simulink model "Modelo_NL_PID_Y_MOD_TORQUE_5_2_2"  (R2017a)
settings: Solver=VariableStepAuto  StartTime=0.0  StopTime=25  MaxStep=1e-4  RelTol=1e-3
undefined symbols (not defined in the file): alfa_cu, ba, beq, Cts, Jeq, ki, Ksa, Ksia, kt, kt_sin_mejora, kw, kw_sin_mejora, LambdaM, Ld, Lq, Pp, r, R0, Rd, Rq, Rsref, Rts_amb, sigbuilder_block, Tamb, Tleq, Tsref
settings Model: Creator=merem  LastModifiedBy=merem

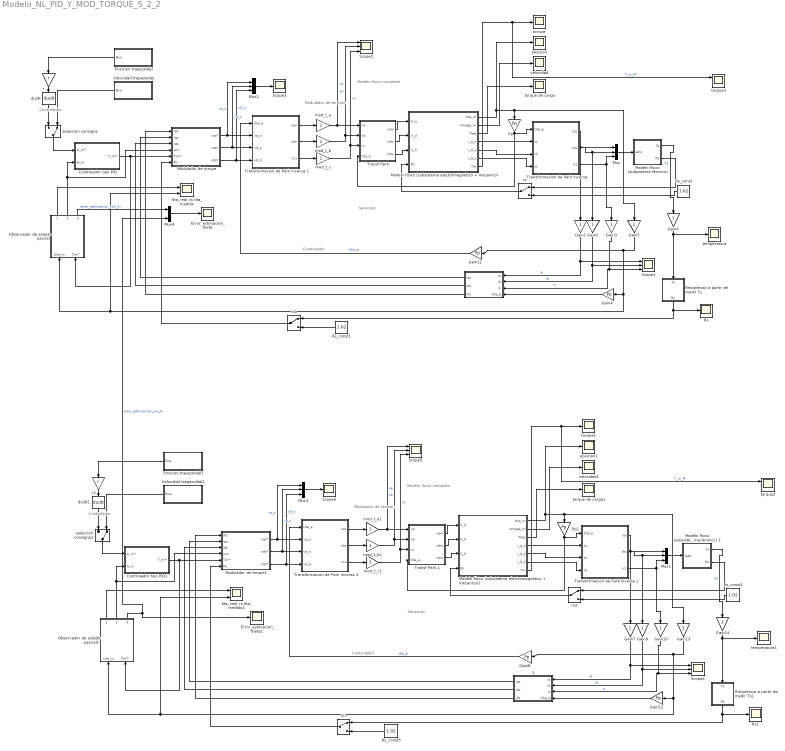
== system Modelo_NL_PID_Y_MOD_TORQUE_5_2_2 ==
  note: Controlador
  note: Controlador
  note: Sensores
  note: Modulador de tensión
  note: Modelo físico completo
  note: Controlador
  note: Controlador
  note: Modulador de tensión
  note: Modelo físico completo
  note: Sensores
  " " : Subsystem
  " 1" : Subsystem
  Controlador tipo PID : Subsystem
  Controlador tipo PID1 : Subsystem
  Error_estimación_theta : Scope
  Error_estimación_theta1 : Scope
  Gain{1..3,5..7,9..10,13..14} (10 alike) : Gain
  Gain{4,8,11..12} (4 alike) : Gain  Gain=Pp
  Modelo físico (subsistema electromagnético + mecanico) : Subsystem
  Modelo físico (subsistema electromagnético + mecanico)1 : Subsystem
  "Modelo físico (subsistema térmico) " : Subsystem
  Modelo físico (subsistema térmico) 1 : Subsystem
  Modulador de torque : Subsystem
  Modulador de torque1 : Subsystem
  Mux{,1..3} (4 alike) : Mux  Inputs=3
  Mux4 : Mux  Inputs=2
  Observador de estado parcial : Subsystem
  Observador de estado parcial1 : Subsystem
  Posicion trapezoidal : Subsystem  Tag=STV Subsys  LoadFcn=sigbuilder_block('load');  StartFcn=sigbuilder_block('start');  StopFcn=sigbuilder_block('stop');  ClipboardFcn=sigbuilder_block('clipboard');  mask(Sigbuilder block){tuvar=[0:10]}
      mask help: Simulink:masks:SigbuilderBlock_MD
      mask init:
      | if ~strcmp(get_param(bdroot(gcbh),'SimulationStatus'),'stopped') tuvar = sigbuilder_block('maskInit'); end
      settings: CopyFcn=sigbuilder_block('copy');  DeleteFcn=sigbuilder_block('delete');  ModelCloseFcn=sigbuilder_block('modelClose');  PreSaveFcn=sigbuilder_block('preSave');  PauseFcn=sigbuilder_block('pause');  ContinueFcn=sigbuilder_block('continue');  NameChangeFcn=sigbuilder_block('namechange');  OpenFcn=sigbuilder_block('open',[6 30 1012.5 447.75 ]);  CloseFcn=sigbuilder_block('close');
      mask Display: plot(0, 0, 100, 100,[2, 2, 32, 32, 2], [68, 8, 8, 68, 68],[32, 2], [38, 38], [32, 19, 2],[53, 60, 44], [32, 17, 17, 2],[16, 16, 31, 31]);txt = getActiveGroup(gcbh);text(2, 100, txt,'verticalAlignment', 'top');
  Posicion trapezoidal1 : Subsystem  Tag=STV Subsys  LoadFcn=sigbuilder_block('load');  StartFcn=sigbuilder_block('start');  StopFcn=sigbuilder_block('stop');  ClipboardFcn=sigbuilder_block('clipboard');  mask(Sigbuilder block){tuvar=[0:10]}
      mask help: Simulink:masks:SigbuilderBlock_MD
      mask init:
      | if ~strcmp(get_param(bdroot(gcbh),'SimulationStatus'),'stopped') tuvar = sigbuilder_block('maskInit'); end
      settings: CopyFcn=sigbuilder_block('copy');  DeleteFcn=sigbuilder_block('delete');  ModelCloseFcn=sigbuilder_block('modelClose');  PreSaveFcn=sigbuilder_block('preSave');  PauseFcn=sigbuilder_block('pause');  ContinueFcn=sigbuilder_block('continue');  NameChangeFcn=sigbuilder_block('namechange');  OpenFcn=sigbuilder_block('open',[6 30 1012.5 447.75 ]);  CloseFcn=sigbuilder_block('close');
      mask Display: plot(0, 0, 100, 100,[2, 2, 32, 32, 2], [68, 8, 8, 68, 68],[32, 2], [38, 38], [32, 19, 2],[53, 60, 44], [32, 17, 17, 2],[16, 16, 31, 31]);txt = getActiveGroup(gcbh);text(2, 100, txt,'verticalAlignment', 'top');
  Pp : Gain  Gain=Pp
  Pp1 : Gain  Gain=Pp
  Resistencia a partir de medir Ts : Subsystem
  Resistencia a partir de medir Ts1 : Subsystem
  Rs : Scope
  Rs1 : Scope
  Rs_const{,1..3} (4 alike) : Constant  Value=1.02
  Scope{1..2,4..5} (4 alike) : Scope  NumInputPorts=3
  Scope3 : Scope
  Scope6 : Scope
  "Transf Park " : Subsystem
  Transf Park 1 : Subsystem
  "Transformacion de Park inversa " : Subsystem
  Transformacion de Park inversa 1 : Subsystem
  Transformacion de Park inversa 2 : Subsystem
  Transformacion de Park inversa 3 : Subsystem
  Velocidad trapezoidal : Subsystem  Tag=STV Subsys  LoadFcn=sigbuilder_block('load');  StartFcn=sigbuilder_block('start');  StopFcn=sigbuilder_block('stop');  ClipboardFcn=sigbuilder_block('clipboard');  mask(Sigbuilder block){tuvar=[0:10]}
      mask help: Simulink:masks:SigbuilderBlock_MD
      mask init:
      | if ~strcmp(get_param(bdroot(gcbh),'SimulationStatus'),'stopped') tuvar = sigbuilder_block('maskInit'); end
      settings: CopyFcn=sigbuilder_block('copy');  DeleteFcn=sigbuilder_block('delete');  ModelCloseFcn=sigbuilder_block('modelClose');  PreSaveFcn=sigbuilder_block('preSave');  PauseFcn=sigbuilder_block('pause');  ContinueFcn=sigbuilder_block('continue');  NameChangeFcn=sigbuilder_block('namechange');  OpenFcn=sigbuilder_block('open',[6 30 1012.5 447.75 ]);  CloseFcn=sigbuilder_block('close');
      mask Display: plot(0, 0, 100, 100,[2, 2, 32, 32, 2], [68, 8, 8, 68, 68],[32, 2], [38, 38], [32, 19, 2],[53, 60, 44], [32, 17, 17, 2],[16, 16, 31, 31]);txt = getActiveGroup(gcbh);text(2, 100, txt,'verticalAlignment', 'top');
  Velocidad trapezoidal1 : Subsystem  Tag=STV Subsys  LoadFcn=sigbuilder_block('load');  StartFcn=sigbuilder_block('start');  StopFcn=sigbuilder_block('stop');  ClipboardFcn=sigbuilder_block('clipboard');  mask(Sigbuilder block){tuvar=[0:10]}
      mask help: Simulink:masks:SigbuilderBlock_MD
      mask init:
      | if ~strcmp(get_param(bdroot(gcbh),'SimulationStatus'),'stopped') tuvar = sigbuilder_block('maskInit'); end
      settings: CopyFcn=sigbuilder_block('copy');  DeleteFcn=sigbuilder_block('delete');  ModelCloseFcn=sigbuilder_block('modelClose');  PreSaveFcn=sigbuilder_block('preSave');  PauseFcn=sigbuilder_block('pause');  ContinueFcn=sigbuilder_block('continue');  NameChangeFcn=sigbuilder_block('namechange');  OpenFcn=sigbuilder_block('open',[6 30 1012.5 447.75 ]);  CloseFcn=sigbuilder_block('close');
      mask Display: plot(0, 0, 100, 100,[2, 2, 32, 32, 2], [68, 8, 8, 68, 68],[32, 2], [38, 38], [32, 19, 2],[53, 60, 44], [32, 17, 17, 2],[16, 16, 31, 31]);txt = getActiveGroup(gcbh);text(2, 100, txt,'verticalAlignment', 'top');
  du/dt : Derivative
  du/dt1 : Derivative
  mod_t_a : Gain
  mod_t_a1 : Gain
  mod_t_b : Gain
  mod_t_b1 : Gain
  mod_t_c : Gain
  mod_t_c1 : Gain
  posicion : Scope
  posicion1 : Scope
  r : Gain  Gain=r
  r1 : Gain  Gain=r
  rs{,1..3} (4 alike) : ManualSwitch
  selección consigna : ManualSwitch  CurrentSetting=0
  selección consigna1 : ManualSwitch  CurrentSetting=0
  temperatura : Scope
  temperatura1 : Scope
  tita_real vs tita_medido : Scope  NumInputPorts=2
  tita_real vs tita_medido1 : Scope  NumInputPorts=2
  torque : Scope
  torque de carga : Scope
  torque de carga1 : Scope
  torque1 : Scope
  torque2 : Scope  NumInputPorts=2
  torque3 : Scope  NumInputPorts=2
  velocidad : Scope
  velocidad1 : Scope
  wires:
  mod_t_c/1 -> Scope2/3, "Transf Park "/3(vc)  "vc"
  Transformacion de Park inversa 1/1(vas) -> mod_t_a/1
  mod_t_a/1 -> Scope2/1, "Transf Park "/1("va ")  "va"
  " "/2("ids ") -> Modulador de torque/3(ids)
  Transformacion de Park inversa 1/3("vcs ") -> mod_t_c/1
  "Modelo físico (subsistema térmico) "/1(Ts) -> Gain6/1  "Ts"
  " "/1(iqs) -> Modulador de torque/2(iqs)
  Transformacion de Park inversa 1/2(vbs) -> mod_t_b/1
  "Transf Park "/2("vdrs ") -> Modelo físico (subsistema electromagnético + mecanico)/2(V_d)
  Mux/1 -> "Modelo físico (subsistema térmico) "/1(iabc)
  Modelo físico (subsistema electromagnético + mecanico)/3(Tleq) -> torque de carga/1
  Gain2/1 -> " "/2("ib "), Scope1/2  "ib"
  Gain3/1 -> " "/3("ic "), Scope1/3  "ic"
  Modelo físico (subsistema electromagnético + mecanico)/1("tita_m ") -> posicion/1, Gain5/1, Pp/1
  mod_t_b/1 -> Scope2/2, "Transf Park "/2(vb)  "vb"
  "Transf Park "/3("v0rs ") -> Modelo físico (subsistema electromagnético + mecanico)/3(V_0)
  Pp/1 -> "Transf Park "/4(tita_e), "Transformacion de Park inversa "/1(tita_e)
  Gain1/1 -> " "/1("ia "), Scope1/1  "ia"
  "Transf Park "/1(vqrs) -> Modelo físico (subsistema electromagnético + mecanico)/1(V_q)
  " "/3("i0s ") -> Modulador de torque/1(i0s)
  Modulador de torque/1(vqs*) -> Transformacion de Park inversa 1/2(vq_s), Mux2/1  "vq_s"
  Modulador de torque/3(v0s*) -> Transformacion de Park inversa 1/4("v0_S "), Mux2/3  "v0_s"
  Modulador de torque/2(vds*) -> Transformacion de Park inversa 1/3(vd_s), Mux2/2  "vd_s"
  Gain11/1 -> Transformacion de Park inversa 1/1(tita_e)  "tita_e"
  Observador de estado parcial/2(w_m_obs) -> Controlador tipo PID/2(w_m), Modulador de torque/4(wm)
  Observador de estado parcial/1("tita_obs ") -> tita_real vs tita_medido/1
  Gain5/1 -> Observador de estado parcial/1(tita_m), tita_real vs tita_medido/2, Gain4/1, Gain11/1
  r/1 -> du/dt/1
  Posicion trapezoidal/1(Bus) -> r/1
  Controlador tipo PID/1(T_m*') -> Observador de estado parcial/2(Tm*'), Modulador de torque/5(Tm*')
  Mux2/1 -> Scope3/1
  Modelo físico (subsistema electromagnético + mecanico)/4("i_q_s ") -> "Transformacion de Park inversa "/2(iq)
  Modelo físico (subsistema electromagnético + mecanico)/5("i_d_s ") -> "Transformacion de Park inversa "/3(id)
  Modelo físico (subsistema electromagnético + mecanico)/6("i_0_s ") -> "Transformacion de Park inversa "/4(i0)
  "Transformacion de Park inversa "/3("ics ") -> Gain3/1, Mux/3
  "Transformacion de Park inversa "/2(ibs) -> Gain2/1, Mux/2
  "Transformacion de Park inversa "/1(ias) -> Gain1/1, Mux/1
  Gain4/1 -> " "/4("tita_e ")
  selección consigna/1 -> Controlador tipo PID/1(w_m*)
  du/dt/1 -> selección consigna/1
  Velocidad trapezoidal/1(Bus) -> selección consigna/2
  Gain6/1 -> temperatura/1, Resistencia a partir de medir Ts/1(Ts)
  Rs_const/1 -> rs/2
  rs/1 -> Modelo físico (subsistema electromagnético + mecanico)/4(Rs)
  "Modelo físico (subsistema térmico) "/2(Rs) -> rs/1
  Modelo físico (subsistema electromagnético + mecanico)/7(Tm) -> torque3/1, torque/1  "T_m_ff"
  rs1/1 -> Modulador de torque/6(Rs)
  Resistencia a partir de medir Ts/1(Rs) -> rs1/1, Rs/1
  Rs_const1/1 -> rs1/2
  Modelo físico (subsistema electromagnético + mecanico)/2("omega_m ") -> velocidad/1
  Mux4/1 -> Error_estimación_theta/1
  Observador de estado parcial/3(error_estim) -> Mux4/1  "error_estimacion_con_ki"
  Gain14/1 -> temperatura1/1, Resistencia a partir de medir Ts1/1(Ts)
  Gain13/1 -> Observador de estado parcial1/1(tita_m), tita_real vs tita_medido1/2, Gain12/1, Gain8/1
  Gain10/1 -> " 1"/3("ic "), Scope4/3  "ic"
  Gain7/1 -> " 1"/1("ia "), Scope4/1  "ia"
  Gain9/1 -> " 1"/2("ib "), Scope4/2  "ib"
  Rs_const3/1 -> rs3/2
  Modelo físico (subsistema electromagnético + mecanico)1/2("omega_m ") -> velocidad1/1
  Modelo físico (subsistema electromagnético + mecanico)1/3(Tleq) -> torque de carga1/1
  Observador de estado parcial1/3(error_estim) -> Error_estimación_theta1/1, Mux4/2  "error_estimacion_sin_ki"
  Resistencia a partir de medir Ts1/1(Rs) -> rs3/1, Rs1/1
  Transformacion de Park inversa 3/1(vas) -> mod_t_a1/1
  Modulador de torque1/3(v0s*) -> Transformacion de Park inversa 3/4("v0_S "), Mux3/3  "v0_s"
  Gain12/1 -> " 1"/4("tita_e ")
  Modelo físico (subsistema térmico) 1/2(Rs) -> rs2/1
  Modelo físico (subsistema electromagnético + mecanico)1/7(Tm) -> torque2/1, torque1/1  "T_m_ff"
  rs3/1 -> Modulador de torque1/6(Rs)
  Transf Park 1/1(vqrs) -> Modelo físico (subsistema electromagnético + mecanico)1/1(V_q)
  Transformacion de Park inversa 2/2(ibs) -> Gain9/1, Mux1/2
  Transformacion de Park inversa 3/3("vcs ") -> mod_t_c1/1
  Transformacion de Park inversa 2/1(ias) -> Gain7/1, Mux1/1
  rs2/1 -> Modelo físico (subsistema electromagnético + mecanico)1/4(Rs)
  Rs_const2/1 -> rs2/2
  Posicion trapezoidal1/1(Bus) -> r1/1
  Velocidad trapezoidal1/1(Bus) -> selección consigna1/2
  Pp1/1 -> Transf Park 1/4(tita_e), Transformacion de Park inversa 2/1(tita_e)
  mod_t_c1/1 -> Scope5/3, Transf Park 1/3(vc)  "vc"
  selección consigna1/1 -> Controlador tipo PID1/1(w_m*)
  Transf Park 1/2("vdrs ") -> Modelo físico (subsistema electromagnético + mecanico)1/2(V_d)
  r1/1 -> du/dt1/1
  Controlador tipo PID1/1(T_m*') -> Observador de estado parcial1/2(Tm*'), Modulador de torque1/5(Tm*')
  Observador de estado parcial1/2(w_m_obs) -> Controlador tipo PID1/2(w_m), Modulador de torque1/4(wm)
  Observador de estado parcial1/1("tita_obs ") -> tita_real vs tita_medido1/1
  Mux1/1 -> Modelo físico (subsistema térmico) 1/1(iabc)
  Modulador de torque1/2(vds*) -> Transformacion de Park inversa 3/3(vd_s), Mux3/2  "vd_s"
  du/dt1/1 -> selección consigna1/1
  mod_t_b1/1 -> Scope5/2, Transf Park 1/2(vb)  "vb"
  " 1"/3("i0s ") -> Modulador de torque1/1(i0s)
  Modulador de torque1/1(vqs*) -> Transformacion de Park inversa 3/2(vq_s), Mux3/1  "vq_s"
  Transformacion de Park inversa 2/3("ics ") -> Gain10/1, Mux1/3
  Modelo físico (subsistema electromagnético + mecanico)1/4("i_q_s ") -> Transformacion de Park inversa 2/2(iq)
  Modelo físico (subsistema electromagnético + mecanico)1/6("i_0_s ") -> Transformacion de Park inversa 2/4(i0)
  " 1"/1(iqs) -> Modulador de torque1/2(iqs)
  Transformacion de Park inversa 3/2(vbs) -> mod_t_b1/1
  Modelo físico (subsistema térmico) 1/1(Ts) -> Gain14/1  "Ts"
  Gain8/1 -> Transformacion de Park inversa 3/1(tita_e)  "tita_e"
  Transf Park 1/3("v0rs ") -> Modelo físico (subsistema electromagnético + mecanico)1/3(V_0)
  Modelo físico (subsistema electromagnético + mecanico)1/1("tita_m ") -> posicion1/1, Gain13/1, Pp1/1
  " 1"/2("ids ") -> Modulador de torque1/3(ids)
  Modelo físico (subsistema electromagnético + mecanico)1/5("i_d_s ") -> Transformacion de Park inversa 2/3(id)
  Mux3/1 -> Scope6/1
  mod_t_a1/1 -> Scope5/1, Transf Park 1/1("va ")  "va"

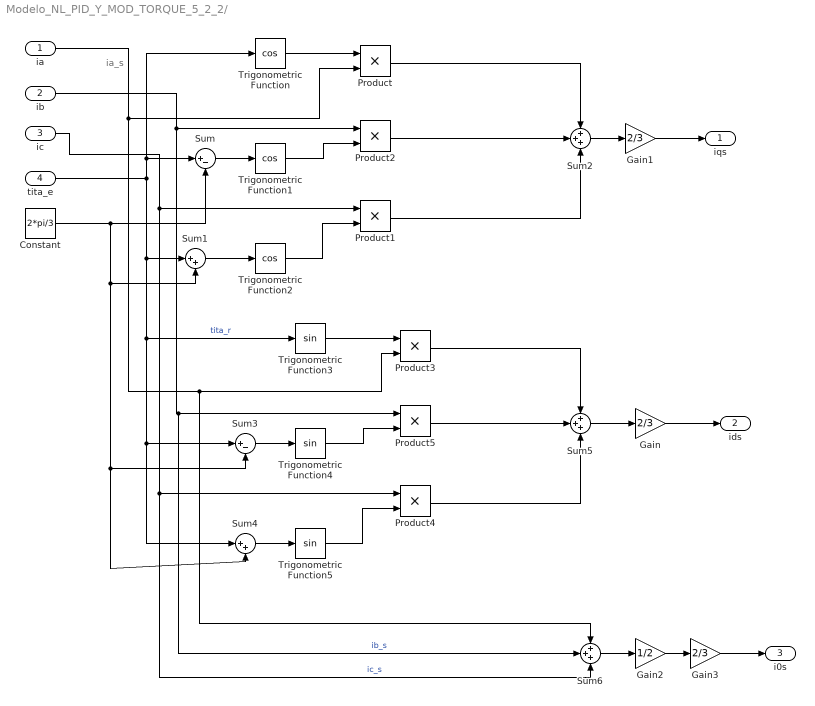
== system Modelo_NL_PID_Y_MOD_TORQUE_5_2_2/  ==
  note: ia_s
  "ia " : Inport
  "ib " : Inport  Port=2
  "ic " : Inport  Port=3
  "tita_e " : Inport  Port=4
  Constant : Constant  Value=2*pi/3
  Gain : Gain  Gain=2/3
  Gain1 : Gain  Gain=2/3
  Gain2 : Gain  Gain=1/2
  Gain3 : Gain  Gain=2/3
  Product{,1..5} (6 alike) : Product
  Sum : Sum  Inputs=|+-
  Sum1 : Sum  Inputs=|++
  Sum2 : Sum  Inputs=+++
  Sum3 : Sum  Inputs=|+-
  Sum4 : Sum  Inputs=|++
  Sum5 : Sum  Inputs=+++
  Sum6 : Sum  Inputs=+++
  Trigonometric Function : Trigonometry  Operator=cos
  Trigonometric Function1 : Trigonometry  Operator=cos
  Trigonometric Function2 : Trigonometry  Operator=cos
  Trigonometric Function3 : Trigonometry
  Trigonometric Function4 : Trigonometry
  Trigonometric Function5 : Trigonometry
  iqs : Outport
  "ids " : Outport  Port=2
  "i0s " : Outport  Port=3
  wires:
  "tita_e "/1 -> Trigonometric Function/1, Sum/1, Sum1/1, Trigonometric Function3/1, Sum3/1, Sum4/1  "tita_r"
  Trigonometric Function/1 -> Product/1
  "ia "/1 -> Sum6/1, Product3/2, Product/2
  Constant/1 -> Sum4/2, Sum3/2, Sum1/2, Sum/2
  Sum/1 -> Trigonometric Function1/1
  Sum1/1 -> Trigonometric Function2/1
  Trigonometric Function1/1 -> Product2/2
  Trigonometric Function2/1 -> Product1/2
  "ib "/1 -> Sum6/2, Product5/1, Product2/1  "ib_s"
  "ic "/1 -> Sum6/3, Product4/1, Product1/1  "ic_s"
  Product/1 -> Sum2/1
  Product2/1 -> Sum2/2
  Sum2/1 -> Gain1/1
  Trigonometric Function5/1 -> Product4/2
  Trigonometric Function3/1 -> Product3/1
  Sum4/1 -> Trigonometric Function5/1
  Sum3/1 -> Trigonometric Function4/1
  Trigonometric Function4/1 -> Product5/2
  Product3/1 -> Sum5/1
  Product5/1 -> Sum5/2
  Product4/1 -> Sum5/3
  Sum5/1 -> Gain/1
  Product1/1 -> Sum2/3
  Gain/1 -> "ids "/1
  Gain1/1 -> iqs/1
  Sum6/1 -> Gain2/1
  Gain2/1 -> Gain3/1
  Gain3/1 -> "i0s "/1

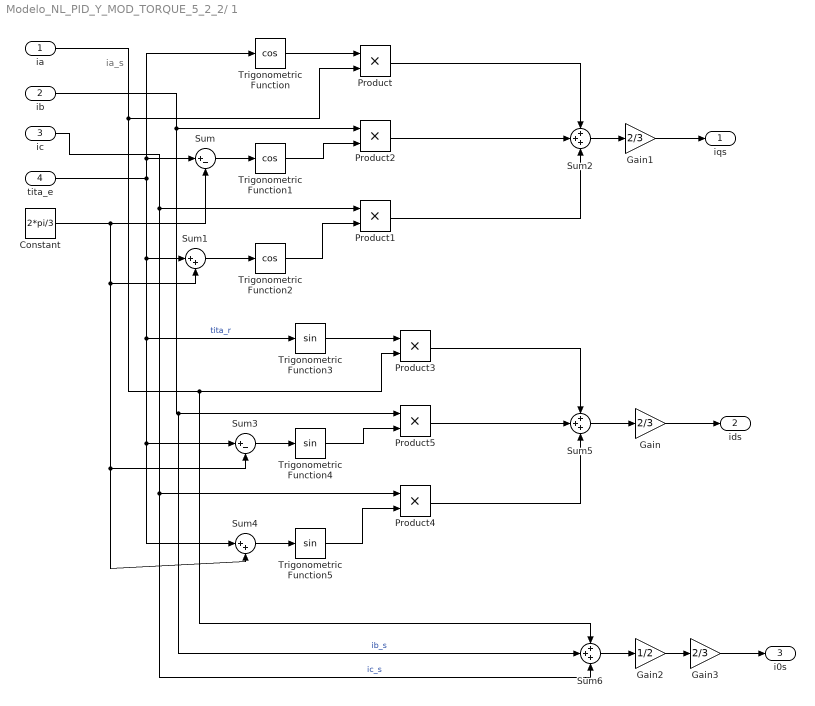
== system Modelo_NL_PID_Y_MOD_TORQUE_5_2_2/ 1 ==
  note: ia_s
  "ia " : Inport
  "ib " : Inport  Port=2
  "ic " : Inport  Port=3
  "tita_e " : Inport  Port=4
  Constant : Constant  Value=2*pi/3
  Gain : Gain  Gain=2/3
  Gain1 : Gain  Gain=2/3
  Gain2 : Gain  Gain=1/2
  Gain3 : Gain  Gain=2/3
  Product{,1..5} (6 alike) : Product
  Sum : Sum  Inputs=|+-
  Sum1 : Sum  Inputs=|++
  Sum2 : Sum  Inputs=+++
  Sum3 : Sum  Inputs=|+-
  Sum4 : Sum  Inputs=|++
  Sum5 : Sum  Inputs=+++
  Sum6 : Sum  Inputs=+++
  Trigonometric Function : Trigonometry  Operator=cos
  Trigonometric Function1 : Trigonometry  Operator=cos
  Trigonometric Function2 : Trigonometry  Operator=cos
  Trigonometric Function3 : Trigonometry
  Trigonometric Function4 : Trigonometry
  Trigonometric Function5 : Trigonometry
  iqs : Outport
  "ids " : Outport  Port=2
  "i0s " : Outport  Port=3
  wires:
  "tita_e "/1 -> Trigonometric Function/1, Sum/1, Sum1/1, Trigonometric Function3/1, Sum3/1, Sum4/1  "tita_r"
  Trigonometric Function/1 -> Product/1
  "ia "/1 -> Sum6/1, Product3/2, Product/2
  Constant/1 -> Sum4/2, Sum3/2, Sum1/2, Sum/2
  Sum/1 -> Trigonometric Function1/1
  Sum1/1 -> Trigonometric Function2/1
  Trigonometric Function1/1 -> Product2/2
  Trigonometric Function2/1 -> Product1/2
  "ib "/1 -> Sum6/2, Product5/1, Product2/1  "ib_s"
  "ic "/1 -> Sum6/3, Product4/1, Product1/1  "ic_s"
  Product/1 -> Sum2/1
  Product2/1 -> Sum2/2
  Sum2/1 -> Gain1/1
  Trigonometric Function5/1 -> Product4/2
  Trigonometric Function3/1 -> Product3/1
  Sum4/1 -> Trigonometric Function5/1
  Sum3/1 -> Trigonometric Function4/1
  Trigonometric Function4/1 -> Product5/2
  Product3/1 -> Sum5/1
  Product5/1 -> Sum5/2
  Product4/1 -> Sum5/3
  Sum5/1 -> Gain/1
  Product1/1 -> Sum2/3
  Gain/1 -> "ids "/1
  Gain1/1 -> iqs/1
  Sum6/1 -> Gain2/1
  Gain2/1 -> Gain3/1
  Gain3/1 -> "i0s "/1

== system Modelo_NL_PID_Y_MOD_TORQUE_5_2_2/Controlador tipo PID ==
  w_m* : Inport
  w_m : Inport  Port=2
  Integrator : Integrator
  Integrator1 : Integrator
  Ksa : Gain  Gain=Ksa
  Ksia : Gain  Gain=Ksia
  Sum : Sum  Inputs=|+-
  Sum1 : Sum  Inputs=+++
  ba : Gain  Gain=ba
  T_m*' : Outport
  wires:
  w_m*/1 -> Sum/1
  w_m/1 -> Sum/2
  Sum/1 -> ba/1, Integrator/1
  Integrator/1 -> Integrator1/1, Ksa/1
  Ksa/1 -> Sum1/2
  ba/1 -> Sum1/3
  Ksia/1 -> Sum1/1
  Sum1/1 -> T_m*'/1
  Integrator1/1 -> Ksia/1

== system Modelo_NL_PID_Y_MOD_TORQUE_5_2_2/Controlador tipo PID1 ==
  w_m* : Inport
  w_m : Inport  Port=2
  Integrator : Integrator
  Integrator1 : Integrator
  Ksa : Gain  Gain=Ksa
  Ksia : Gain  Gain=Ksia
  Sum : Sum  Inputs=|+-
  Sum1 : Sum  Inputs=+++
  ba : Gain  Gain=ba
  T_m*' : Outport
  wires:
  w_m*/1 -> Sum/1
  w_m/1 -> Sum/2
  Sum/1 -> ba/1, Integrator/1
  Integrator/1 -> Integrator1/1, Ksa/1
  Ksa/1 -> Sum1/2
  ba/1 -> Sum1/3
  Ksia/1 -> Sum1/1
  Sum1/1 -> T_m*'/1
  Integrator1/1 -> Ksia/1

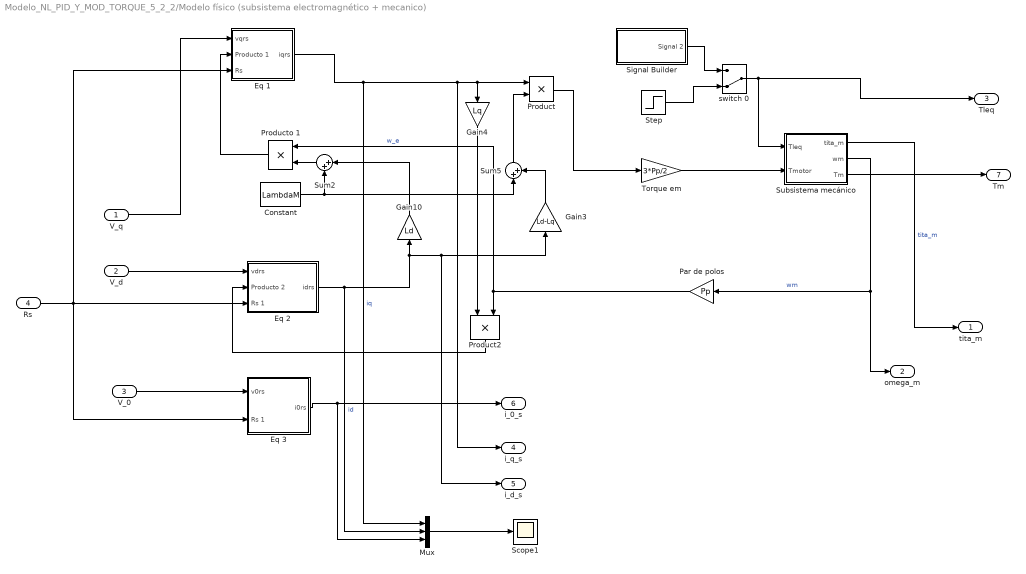
== system Modelo_NL_PID_Y_MOD_TORQUE_5_2_2/Modelo físico (subsistema electromagnético + mecanico) ==
  V_q : Inport
  V_d : Inport  Port=2
  V_0 : Inport  Port=3
  Rs : Inport  Port=4
  Constant : Constant  Value=LambdaM
  Eq 1 : Subsystem
  "Eq 2 " : Subsystem
  Eq 3 : Subsystem
  Gain10 : Gain  Gain=Ld
  Gain3 : Gain  Gain=Ld-Lq
  Gain4 : Gain  Gain=Lq
  Mux : Mux  Inputs=3
  Par de polos : Gain  Gain=Pp
  Product : Product
  Product2 : Product
  Producto 1 : Product
  Scope1 : Scope
  Signal Builder : Subsystem  Tag=STV Subsys  LoadFcn=sigbuilder_block('load');  StartFcn=sigbuilder_block('start');  StopFcn=sigbuilder_block('stop');  ClipboardFcn=sigbuilder_block('clipboard');  mask(Sigbuilder block){tuvar=[0:10]}
      mask help: Simulink:masks:SigbuilderBlock_MD
      mask init:
      | if ~strcmp(get_param(bdroot(gcbh),'SimulationStatus'),'stopped') tuvar = sigbuilder_block('maskInit'); end
      settings: CopyFcn=sigbuilder_block('copy');  DeleteFcn=sigbuilder_block('delete');  ModelCloseFcn=sigbuilder_block('modelClose');  PreSaveFcn=sigbuilder_block('preSave');  PauseFcn=sigbuilder_block('pause');  ContinueFcn=sigbuilder_block('continue');  NameChangeFcn=sigbuilder_block('namechange');  OpenFcn=sigbuilder_block('open',[6 30 1012.5 447.75 ]);  CloseFcn=sigbuilder_block('close');
      mask Display: plot(0, 0, 100, 100,[2, 2, 32, 32, 2], [68, 8, 8, 68, 68],[32, 2], [38, 38], [32, 19, 2],[53, 60, 44], [32, 17, 17, 2],[16, 16, 31, 31]);txt = getActiveGroup(gcbh);text(2, 100, txt,'verticalAlignment', 'top');
  Step : Step  Time=0.3  After=Tleq  SampleTime=0
  Subsistema mecánico : Subsystem
  Sum2 : Sum  Inputs=|++
  Sum5 : Sum  Inputs=|++
  "Torque em " : Gain  Gain=3*Pp/2
  switch 0 : ManualSwitch  CurrentSetting=0
  "tita_m " : Outport
  "omega_m " : Outport  Port=2
  Tleq : Outport  Port=3
  "i_q_s " : Outport  Port=4
  "i_d_s " : Outport  Port=5
  "i_0_s " : Outport  Port=6
  Tm : Outport  Port=7
  wires:
  Sum2/1 -> Producto 1/2
  Sum5/1 -> Product/2
  Subsistema mecánico/2("wm ") -> "omega_m "/1, Par de polos/1  "wm"
  V_q/1 -> Eq 1/1(vqrs)
  Gain10/1 -> Sum2/1
  Par de polos/1 -> Producto 1/1, Product2/2  "w_e"
  "Torque em "/1 -> Subsistema mecánico/2("Tmotor ")
  Product/1 -> "Torque em "/1
  Constant/1 -> Sum5/1, Sum2/2
  Gain3/1 -> Sum5/2
  Gain4/1 -> Product2/1
  Eq 1/1("iqrs ") -> Mux/1, "i_q_s "/1, Gain4/1, Product/1  "iq"
  Subsistema mecánico/1("tita_m ") -> "tita_m "/1  "tita_m"
  "Eq 2 "/1("idrs ") -> Mux/2, "i_d_s "/1, Gain3/1, Gain10/1  "id"
  Product2/1 -> "Eq 2 "/2("Producto 2 ")
  Producto 1/1 -> Eq 1/2("Producto 1 ")
  V_d/1 -> "Eq 2 "/1("vdrs ")
  V_0/1 -> Eq 3/1("v0rs ")
  Eq 3/1("i0rs ") -> Mux/3, "i_0_s "/1
  Step/1 -> switch 0/2
  switch 0/1 -> Subsistema mecánico/1("Tleq "), Tleq/1
  Signal Builder/1(Signal 2) -> switch 0/1
  Rs/1 -> "Eq 2 "/3(Rs 1), Eq 3/2(Rs 1), Eq 1/3(Rs)
  Mux/1 -> Scope1/1
  Subsistema mecánico/3(Tm) -> Tm/1

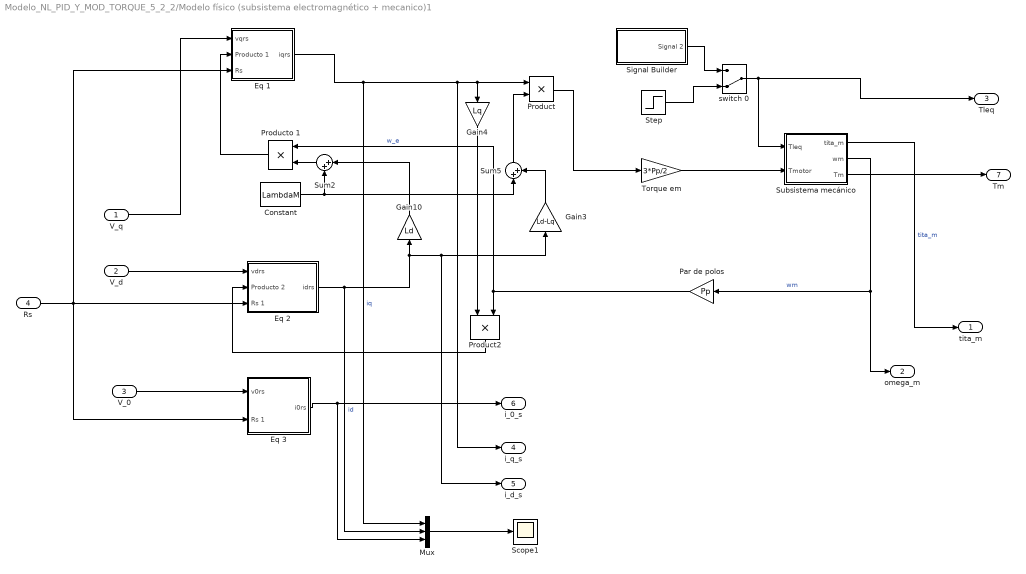
== system Modelo_NL_PID_Y_MOD_TORQUE_5_2_2/Modelo físico (subsistema electromagnético + mecanico)1 ==
  V_q : Inport
  V_d : Inport  Port=2
  V_0 : Inport  Port=3
  Rs : Inport  Port=4
  Constant : Constant  Value=LambdaM
  Eq 1 : Subsystem
  "Eq 2 " : Subsystem
  Eq 3 : Subsystem
  Gain10 : Gain  Gain=Ld
  Gain3 : Gain  Gain=Ld-Lq
  Gain4 : Gain  Gain=Lq
  Mux : Mux  Inputs=3
  Par de polos : Gain  Gain=Pp
  Product : Product
  Product2 : Product
  Producto 1 : Product
  Scope1 : Scope
  Signal Builder : Subsystem  Tag=STV Subsys  LoadFcn=sigbuilder_block('load');  StartFcn=sigbuilder_block('start');  StopFcn=sigbuilder_block('stop');  ClipboardFcn=sigbuilder_block('clipboard');  mask(Sigbuilder block){tuvar=[0:10]}
      mask help: Simulink:masks:SigbuilderBlock_MD
      mask init:
      | if ~strcmp(get_param(bdroot(gcbh),'SimulationStatus'),'stopped') tuvar = sigbuilder_block('maskInit'); end
      settings: CopyFcn=sigbuilder_block('copy');  DeleteFcn=sigbuilder_block('delete');  ModelCloseFcn=sigbuilder_block('modelClose');  PreSaveFcn=sigbuilder_block('preSave');  PauseFcn=sigbuilder_block('pause');  ContinueFcn=sigbuilder_block('continue');  NameChangeFcn=sigbuilder_block('namechange');  OpenFcn=sigbuilder_block('open',[6 30 1012.5 447.75 ]);  CloseFcn=sigbuilder_block('close');
      mask Display: plot(0, 0, 100, 100,[2, 2, 32, 32, 2], [68, 8, 8, 68, 68],[32, 2], [38, 38], [32, 19, 2],[53, 60, 44], [32, 17, 17, 2],[16, 16, 31, 31]);txt = getActiveGroup(gcbh);text(2, 100, txt,'verticalAlignment', 'top');
  Step : Step  Time=0.3  After=Tleq  SampleTime=0
  Subsistema mecánico : Subsystem
  Sum2 : Sum  Inputs=|++
  Sum5 : Sum  Inputs=|++
  "Torque em " : Gain  Gain=3*Pp/2
  switch 0 : ManualSwitch  CurrentSetting=0
  "tita_m " : Outport
  "omega_m " : Outport  Port=2
  Tleq : Outport  Port=3
  "i_q_s " : Outport  Port=4
  "i_d_s " : Outport  Port=5
  "i_0_s " : Outport  Port=6
  Tm : Outport  Port=7
  wires:
  Sum2/1 -> Producto 1/2
  Sum5/1 -> Product/2
  Subsistema mecánico/2("wm ") -> "omega_m "/1, Par de polos/1  "wm"
  V_q/1 -> Eq 1/1(vqrs)
  Gain10/1 -> Sum2/1
  Par de polos/1 -> Producto 1/1, Product2/2  "w_e"
  "Torque em "/1 -> Subsistema mecánico/2("Tmotor ")
  Product/1 -> "Torque em "/1
  Constant/1 -> Sum5/1, Sum2/2
  Gain3/1 -> Sum5/2
  Gain4/1 -> Product2/1
  Eq 1/1("iqrs ") -> Mux/1, "i_q_s "/1, Gain4/1, Product/1  "iq"
  Subsistema mecánico/1("tita_m ") -> "tita_m "/1  "tita_m"
  "Eq 2 "/1("idrs ") -> Mux/2, "i_d_s "/1, Gain3/1, Gain10/1  "id"
  Product2/1 -> "Eq 2 "/2("Producto 2 ")
  Producto 1/1 -> Eq 1/2("Producto 1 ")
  V_d/1 -> "Eq 2 "/1("vdrs ")
  V_0/1 -> Eq 3/1("v0rs ")
  Eq 3/1("i0rs ") -> Mux/3, "i_0_s "/1
  Step/1 -> switch 0/2
  switch 0/1 -> Subsistema mecánico/1("Tleq "), Tleq/1
  Signal Builder/1(Signal 2) -> switch 0/1
  Rs/1 -> "Eq 2 "/3(Rs 1), Eq 3/2(Rs 1), Eq 1/3(Rs)
  Mux/1 -> Scope1/1
  Subsistema mecánico/3(Tm) -> Tm/1

== system Modelo_NL_PID_Y_MOD_TORQUE_5_2_2/Modelo físico (subsistema térmico)  ==
  note: ib
  iabc : Inport
  Constant : Constant  Value=Tsref
  Constant1 : Constant
  Demux : Demux  Outputs=3
  Gain : Gain  Gain=1/Cts
  Gain1 : Gain  Gain=1/Rts_amb
  Gain2 : Gain  Gain=alfa_cu
  Gain3 : Gain  Gain=Rsref
  Integrator : Integrator  InitialCondition=40
  Product{,1..3} (4 alike) : Product
  Sum : Sum  Inputs=+++
  Sum1 : Sum  Inputs=|+-
  Sum2 : Sum  Inputs=|+-
  Sum3 : Sum  Inputs=|++
  Sum4 : Sum  Inputs=|-+
  Tamb 1 : Constant  Value=Tamb
  Ts : Outport
  Rs : Outport  Port=2
  wires:
  iabc/1 -> Demux/1
  Demux/1 -> Product/2, Product/1  "ia"
  Demux/2 -> Product1/2, Product1/1
  Demux/3 -> Product2/2, Product2/1  "ic"
  Product/1 -> Sum/1
  Product1/1 -> Sum/2
  Product2/1 -> Sum/3
  Sum/1 -> Product3/1
  Gain/1 -> Integrator/1
  Product3/1 -> Sum1/1
  Sum1/1 -> Gain/1
  Gain1/1 -> Sum1/2
  Integrator/1 -> Ts/1, Sum4/2, Sum2/1  "Ts"
  Constant/1 -> Sum2/2
  Sum2/1 -> Gain2/1
  Gain2/1 -> Sum3/1
  Constant1/1 -> Sum3/2
  Sum3/1 -> Gain3/1
  Gain3/1 -> Rs/1, Product3/2  "Rs"
  Tamb 1/1 -> Sum4/1
  Sum4/1 -> Gain1/1

== system Modelo_NL_PID_Y_MOD_TORQUE_5_2_2/Modelo físico (subsistema térmico) 1 ==
  note: ib
  iabc : Inport
  Constant : Constant  Value=Tsref
  Constant1 : Constant
  Demux : Demux  Outputs=3
  Gain : Gain  Gain=1/Cts
  Gain1 : Gain  Gain=1/Rts_amb
  Gain2 : Gain  Gain=alfa_cu
  Gain3 : Gain  Gain=Rsref
  Integrator : Integrator  InitialCondition=40
  Product{,1..3} (4 alike) : Product
  Sum : Sum  Inputs=+++
  Sum1 : Sum  Inputs=|+-
  Sum2 : Sum  Inputs=|+-
  Sum3 : Sum  Inputs=|++
  Sum4 : Sum  Inputs=|-+
  Tamb 1 : Constant  Value=Tamb
  Ts : Outport
  Rs : Outport  Port=2
  wires:
  iabc/1 -> Demux/1
  Demux/1 -> Product/2, Product/1  "ia"
  Demux/2 -> Product1/2, Product1/1
  Demux/3 -> Product2/2, Product2/1  "ic"
  Product/1 -> Sum/1
  Product1/1 -> Sum/2
  Product2/1 -> Sum/3
  Sum/1 -> Product3/1
  Gain/1 -> Integrator/1
  Product3/1 -> Sum1/1
  Sum1/1 -> Gain/1
  Gain1/1 -> Sum1/2
  Integrator/1 -> Ts/1, Sum4/2, Sum2/1  "Ts"
  Constant/1 -> Sum2/2
  Sum2/1 -> Gain2/1
  Gain2/1 -> Sum3/1
  Constant1/1 -> Sum3/2
  Sum3/1 -> Gain3/1
  Gain3/1 -> Rs/1, Product3/2  "Rs"
  Tamb 1/1 -> Sum4/1
  Sum4/1 -> Gain1/1

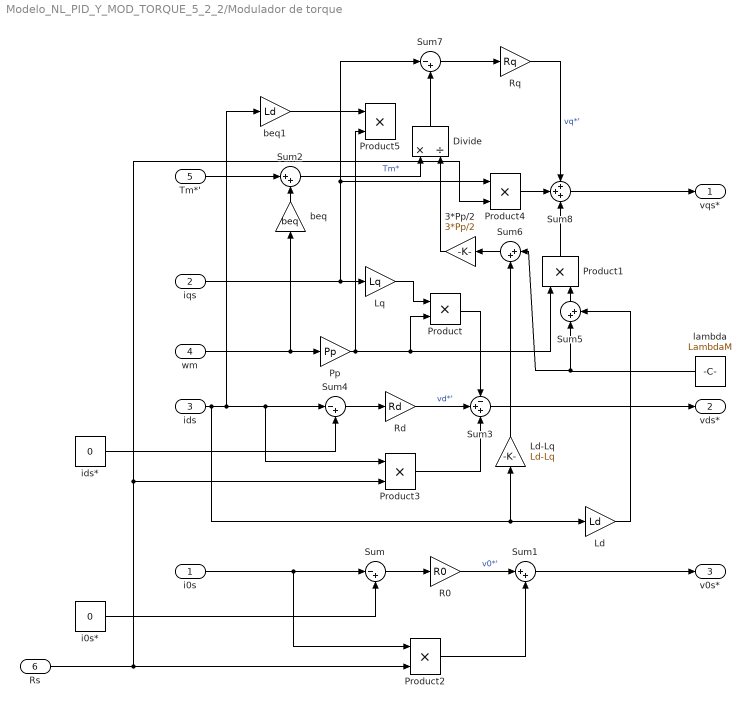
== system Modelo_NL_PID_Y_MOD_TORQUE_5_2_2/Modulador de torque ==
  i0s : Inport
  iqs : Inport  Port=2
  ids : Inport  Port=3
  wm : Inport  Port=4
  Tm*' : Inport  Port=5
  Rs : Inport  Port=6
  3*Pp/2 : Gain  Gain=3*Pp/2
  Divide : Product  Inputs=*/
  Ld : Gain  Gain=Ld
  Ld-Lq : Gain  Gain=Ld-Lq
  Lq : Gain  Gain=Lq
  Pp : Gain  Gain=Pp
  Product{,1..5} (6 alike) : Product
  R0 : Gain  Gain=R0
  Rd : Gain  Gain=Rd
  Rq : Gain  Gain=Rq
  Sum : Sum  Inputs=|-+
  Sum{1..2,5..6} (4 alike) : Sum  Inputs=|++
  Sum3 : Sum  Inputs=-++
  Sum4 : Sum  Inputs=|-+
  Sum7 : Sum  Inputs=|-+
  Sum8 : Sum  Inputs=+++
  beq : Gain  Gain=beq
  beq1 : Gain  Gain=Ld
  i0s* : Constant  Value=0
  ids* : Constant  Value=0
  lambda : Constant  Value=LambdaM
  vqs* : Outport
  vds* : Outport  Port=2
  v0s* : Outport  Port=3
  wires:
  i0s/1 -> Product2/1, Sum/1
  Sum1/1 -> v0s*/1
  Product2/1 -> Sum1/2
  R0/1 -> Sum1/1  "v0*'"
  Sum/1 -> R0/1
  i0s*/1 -> Sum/2
  Sum3/1 -> vds*/1
  Sum4/1 -> Rd/1
  ids/1 -> Ld/1, Ld-Lq/1, beq1/1, Product3/1, Sum4/1
  ids*/1 -> Sum4/2
  wm/1 -> Pp/1, beq/1
  Pp/1 -> Product5/2, Product1/1, Product/2
  iqs/1 -> Product4/1, Sum7/1, Lq/1
  Lq/1 -> Product/1
  Rd/1 -> Sum3/2  "vd*'"
  Product/1 -> Sum3/1
  Tm*'/1 -> Sum2/1
  beq/1 -> Sum2/2
  Ld/1 -> Sum5/2
  lambda/1 -> Sum5/1, Sum6/1
  Sum6/1 -> 3*Pp/2/1
  Sum2/1 -> Divide/1  "Tm*"
  3*Pp/2/1 -> Divide/2
  Sum7/1 -> Rq/1
  Rq/1 -> Sum8/1  "vq*'"
  Product1/1 -> Sum8/3
  Sum8/1 -> vqs*/1
  Product4/1 -> Sum8/2
  Ld-Lq/1 -> Sum6/2
  Product3/1 -> Sum3/3
  Rs/1 -> Product4/2, Product3/2, Product2/2
  Sum5/1 -> Product1/2
  beq1/1 -> Product5/1
  Divide/1 -> Sum7/2

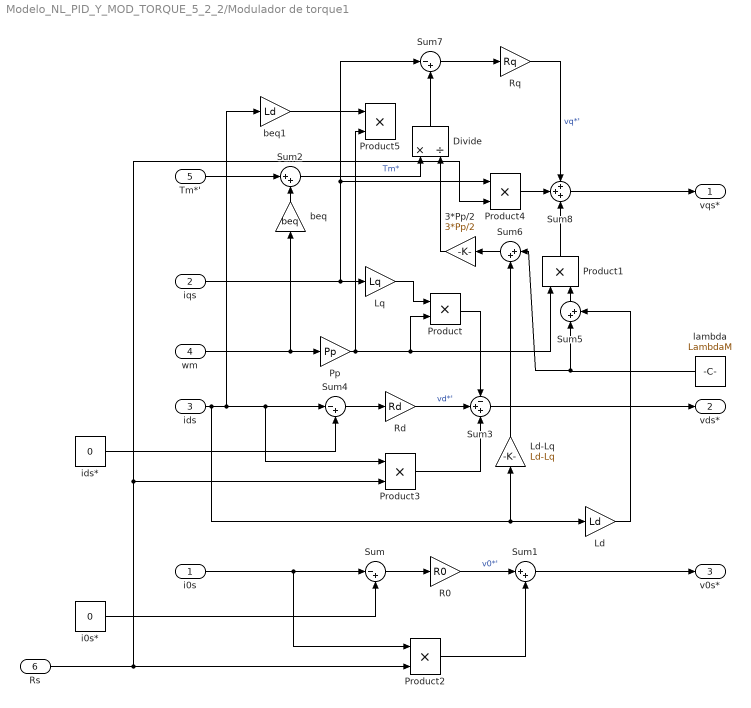
== system Modelo_NL_PID_Y_MOD_TORQUE_5_2_2/Modulador de torque1 ==
  i0s : Inport
  iqs : Inport  Port=2
  ids : Inport  Port=3
  wm : Inport  Port=4
  Tm*' : Inport  Port=5
  Rs : Inport  Port=6
  3*Pp/2 : Gain  Gain=3*Pp/2
  Divide : Product  Inputs=*/
  Ld : Gain  Gain=Ld
  Ld-Lq : Gain  Gain=Ld-Lq
  Lq : Gain  Gain=Lq
  Pp : Gain  Gain=Pp
  Product{,1..5} (6 alike) : Product
  R0 : Gain  Gain=R0
  Rd : Gain  Gain=Rd
  Rq : Gain  Gain=Rq
  Sum : Sum  Inputs=|-+
  Sum{1..2,5..6} (4 alike) : Sum  Inputs=|++
  Sum3 : Sum  Inputs=-++
  Sum4 : Sum  Inputs=|-+
  Sum7 : Sum  Inputs=|-+
  Sum8 : Sum  Inputs=+++
  beq : Gain  Gain=beq
  beq1 : Gain  Gain=Ld
  i0s* : Constant  Value=0
  ids* : Constant  Value=0
  lambda : Constant  Value=LambdaM
  vqs* : Outport
  vds* : Outport  Port=2
  v0s* : Outport  Port=3
  wires:
  i0s/1 -> Product2/1, Sum/1
  Sum1/1 -> v0s*/1
  Product2/1 -> Sum1/2
  R0/1 -> Sum1/1  "v0*'"
  Sum/1 -> R0/1
  i0s*/1 -> Sum/2
  Sum3/1 -> vds*/1
  Sum4/1 -> Rd/1
  ids/1 -> Ld/1, Ld-Lq/1, beq1/1, Product3/1, Sum4/1
  ids*/1 -> Sum4/2
  wm/1 -> Pp/1, beq/1
  Pp/1 -> Product5/2, Product1/1, Product/2
  iqs/1 -> Product4/1, Sum7/1, Lq/1
  Lq/1 -> Product/1
  Rd/1 -> Sum3/2  "vd*'"
  Product/1 -> Sum3/1
  Tm*'/1 -> Sum2/1
  beq/1 -> Sum2/2
  Ld/1 -> Sum5/2
  lambda/1 -> Sum5/1, Sum6/1
  Sum6/1 -> 3*Pp/2/1
  Sum2/1 -> Divide/1  "Tm*"
  3*Pp/2/1 -> Divide/2
  Sum7/1 -> Rq/1
  Rq/1 -> Sum8/1  "vq*'"
  Product1/1 -> Sum8/3
  Sum8/1 -> vqs*/1
  Product4/1 -> Sum8/2
  Ld-Lq/1 -> Sum6/2
  Product3/1 -> Sum3/3
  Rs/1 -> Product4/2, Product3/2, Product2/2
  Sum5/1 -> Product1/2
  beq1/1 -> Product5/1
  Divide/1 -> Sum7/2

== system Modelo_NL_PID_Y_MOD_TORQUE_5_2_2/Observador de estado parcial ==
  tita_m : Inport
  Tm*' : Inport  Port=2
  Gain : Gain  Gain=1/Jeq
  Gain1 : Gain  Gain=kw
  Gain2 : Gain  Gain=kt
  Gain3 : Gain  Gain=ki
  Integrator : Integrator
  Integrator1 : Integrator
  Integrator2 : Integrator
  Sum1 : Sum  Inputs=++|
  Sum2 : Sum  Inputs=+-
  Sum3 : Sum  Inputs=++|
  Sum4 : Sum  Inputs=++|
  "tita_obs " : Outport
  w_m_obs : Outport  Port=2
  error_estim : Outport  Port=3
  wires:
  Sum3/1 -> Integrator/1
  Integrator1/1 -> "tita_obs "/1, Sum2/2
  tita_m/1 -> Sum2/1
  Sum2/1 -> error_estim/1, Gain2/1, Gain3/1, Gain1/1
  Gain2/1 -> Sum1/1
  Integrator/1 -> Sum1/2
  Gain1/1 -> Sum3/1
  Sum1/1 -> w_m_obs/1, Integrator1/1
  Gain3/1 -> Integrator2/1
  Sum4/1 -> Sum3/2
  Tm*'/1 -> Gain/1
  Integrator2/1 -> Sum4/1
  Gain/1 -> Sum4/2

== system Modelo_NL_PID_Y_MOD_TORQUE_5_2_2/Observador de estado parcial1 ==
  tita_m : Inport
  Tm*' : Inport  Port=2
  Gain : Gain  Gain=1/Jeq
  Gain1 : Gain  Gain=kw_sin_mejora
  Gain2 : Gain  Gain=kt_sin_mejora
  Integrator : Integrator
  Integrator1 : Integrator
  Sum1 : Sum  Inputs=++|
  Sum2 : Sum  Inputs=+-
  Sum3 : Sum  Inputs=++|
  "tita_obs " : Outport
  w_m_obs : Outport  Port=2
  error_estim : Outport  Port=3
  wires:
  Sum3/1 -> Integrator/1
  Integrator1/1 -> "tita_obs "/1, Sum2/2
  tita_m/1 -> Sum2/1
  Sum2/1 -> error_estim/1, Gain2/1, Gain1/1
  Gain2/1 -> Sum1/1
  Integrator/1 -> Sum1/2
  Gain1/1 -> Sum3/1
  Sum1/1 -> w_m_obs/1, Integrator1/1
  Tm*'/1 -> Gain/1
  Gain/1 -> Sum3/2

== system Modelo_NL_PID_Y_MOD_TORQUE_5_2_2/Posicion trapezoidal ==
  Bus Creator : BusCreator  Tag=Bus Creator  Inputs=1
  FromWs : FromWorkspace  Tag=STV FromWs  VariableName=tuvar  SampleTime=0
      SigBuilderData=|
      | common.afterFinalStr = 'Extrapolate'
      | common.sampleTime = 0
      | dataSet.timeRange = [0 25]
      | dataSet.name = 'Group 1'
      | sbobj.Groups.Name = 'Group 1'
      | sbobj.Groups.Signals.Name = 'Signal 2'
      | sbobj.Groups.Signals.XData = [0 4 5 10 15 20 25]
      | sbobj.Groups.Signals.YData = [0 0 0 6.28 6.28 0 0]
      | sbobj.Groups.TimeRange = [0 25]
  Subsystem : Subsystem
  Bus : Outport
  wires:
  FromWs/1 -> Subsystem/1(In1)
  Bus Creator/1 -> Bus/1
  Subsystem/1(Signal 2) -> Bus Creator/1  "Signal 2"

== system Modelo_NL_PID_Y_MOD_TORQUE_5_2_2/Posicion trapezoidal1 ==
  Bus Creator : BusCreator  Tag=Bus Creator  Inputs=1
  FromWs : FromWorkspace  Tag=STV FromWs  VariableName=tuvar  SampleTime=0
      SigBuilderData=|
      | common.afterFinalStr = 'Extrapolate'
      | common.sampleTime = 0
      | dataSet.timeRange = [0 25]
      | dataSet.name = 'Group 1'
      | sbobj.Groups.Name = 'Group 1'
      | sbobj.Groups.Signals.Name = 'Signal 2'
      | sbobj.Groups.Signals.XData = [0 4 5 10 15 20 25]
      | sbobj.Groups.Signals.YData = [0 0 0 6.28 6.28 0 0]
      | sbobj.Groups.TimeRange = [0 25]
  Subsystem : Subsystem
  Bus : Outport
  wires:
  FromWs/1 -> Subsystem/1(In1)
  Bus Creator/1 -> Bus/1
  Subsystem/1(Signal 2) -> Bus Creator/1  "Signal 2"

== system Modelo_NL_PID_Y_MOD_TORQUE_5_2_2/Resistencia a partir de medir Ts ==
  Ts : Inport
  Constant2 : Constant  Value=Tsref
  Constant3 : Constant
  Gain4 : Gain  Gain=alfa_cu
  Gain5 : Gain  Gain=Rsref
  Sum5 : Sum  Inputs=|+-
  Sum6 : Sum  Inputs=|++
  Rs : Outport
  wires:
  Constant3/1 -> Sum6/2
  Sum5/1 -> Gain4/1
  Gain5/1 -> Rs/1  "Rs"
  Constant2/1 -> Sum5/2
  Gain4/1 -> Sum6/1
  Sum6/1 -> Gain5/1
  Ts/1 -> Sum5/1

== system Modelo_NL_PID_Y_MOD_TORQUE_5_2_2/Resistencia a partir de medir Ts1 ==
  Ts : Inport
  Constant2 : Constant  Value=Tsref
  Constant3 : Constant
  Gain4 : Gain  Gain=alfa_cu
  Gain5 : Gain  Gain=Rsref
  Sum5 : Sum  Inputs=|+-
  Sum6 : Sum  Inputs=|++
  Rs : Outport
  wires:
  Constant3/1 -> Sum6/2
  Sum5/1 -> Gain4/1
  Gain5/1 -> Rs/1  "Rs"
  Constant2/1 -> Sum5/2
  Gain4/1 -> Sum6/1
  Sum6/1 -> Gain5/1
  Ts/1 -> Sum5/1

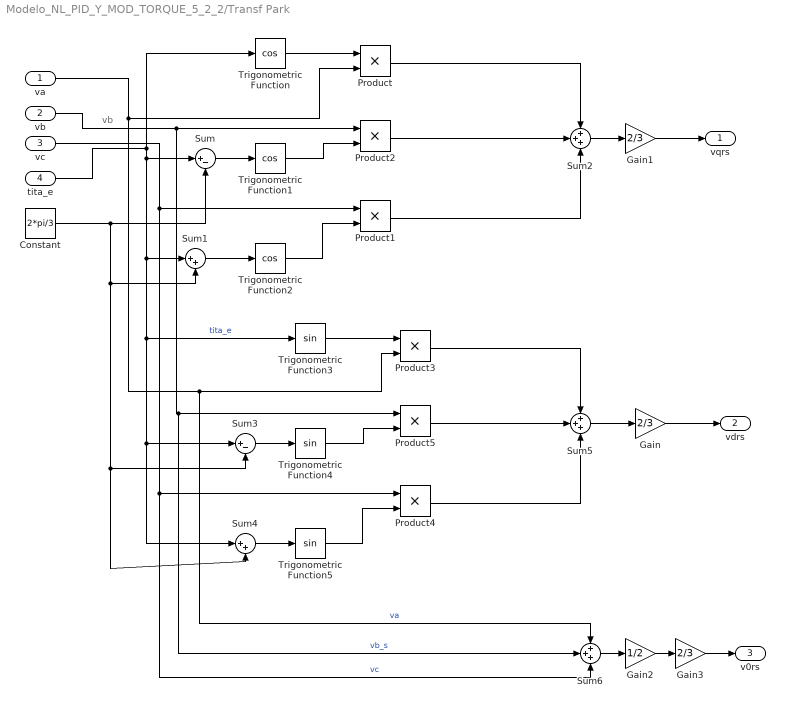
== system Modelo_NL_PID_Y_MOD_TORQUE_5_2_2/Transf Park  ==
  note: vb
  "va " : Inport
  vb : Inport  Port=2
  vc : Inport  Port=3
  tita_e : Inport  Port=4
  Constant : Constant  Value=2*pi/3
  Gain : Gain  Gain=2/3
  Gain1 : Gain  Gain=2/3
  Gain2 : Gain  Gain=1/2
  Gain3 : Gain  Gain=2/3
  Product{,1..5} (6 alike) : Product
  Sum : Sum  Inputs=|+-
  Sum1 : Sum  Inputs=|++
  Sum2 : Sum  Inputs=+++
  Sum3 : Sum  Inputs=|+-
  Sum4 : Sum  Inputs=|++
  Sum5 : Sum  Inputs=+++
  Sum6 : Sum  Inputs=+++
  Trigonometric Function : Trigonometry  Operator=cos
  Trigonometric Function1 : Trigonometry  Operator=cos
  Trigonometric Function2 : Trigonometry  Operator=cos
  Trigonometric Function3 : Trigonometry
  Trigonometric Function4 : Trigonometry
  Trigonometric Function5 : Trigonometry
  vqrs : Outport
  "vdrs " : Outport  Port=2
  "v0rs " : Outport  Port=3
  wires:
  tita_e/1 -> Sum1/1, Trigonometric Function3/1, Sum3/1, Sum4/1, Sum/1, Trigonometric Function/1  "tita_e"
  Trigonometric Function/1 -> Product/1
  "va "/1 -> Sum6/1, Product3/2, Product/2  "va"
  Constant/1 -> Sum4/2, Sum3/2, Sum1/2, Sum/2
  Sum/1 -> Trigonometric Function1/1
  Sum1/1 -> Trigonometric Function2/1
  Trigonometric Function1/1 -> Product2/2
  Trigonometric Function2/1 -> Product1/2
  vb/1 -> Sum6/2, Product5/1, Product2/1  "vb_s"
  vc/1 -> Sum6/3, Product4/1, Product1/1  "vc"
  Product/1 -> Sum2/1
  Product2/1 -> Sum2/2
  Sum2/1 -> Gain1/1
  Trigonometric Function5/1 -> Product4/2
  Trigonometric Function3/1 -> Product3/1
  Sum4/1 -> Trigonometric Function5/1
  Sum3/1 -> Trigonometric Function4/1
  Trigonometric Function4/1 -> Product5/2
  Product3/1 -> Sum5/1
  Product5/1 -> Sum5/2
  Product4/1 -> Sum5/3
  Sum5/1 -> Gain/1
  Product1/1 -> Sum2/3
  Gain/1 -> "vdrs "/1
  Gain1/1 -> vqrs/1
  Sum6/1 -> Gain2/1
  Gain3/1 -> "v0rs "/1
  Gain2/1 -> Gain3/1

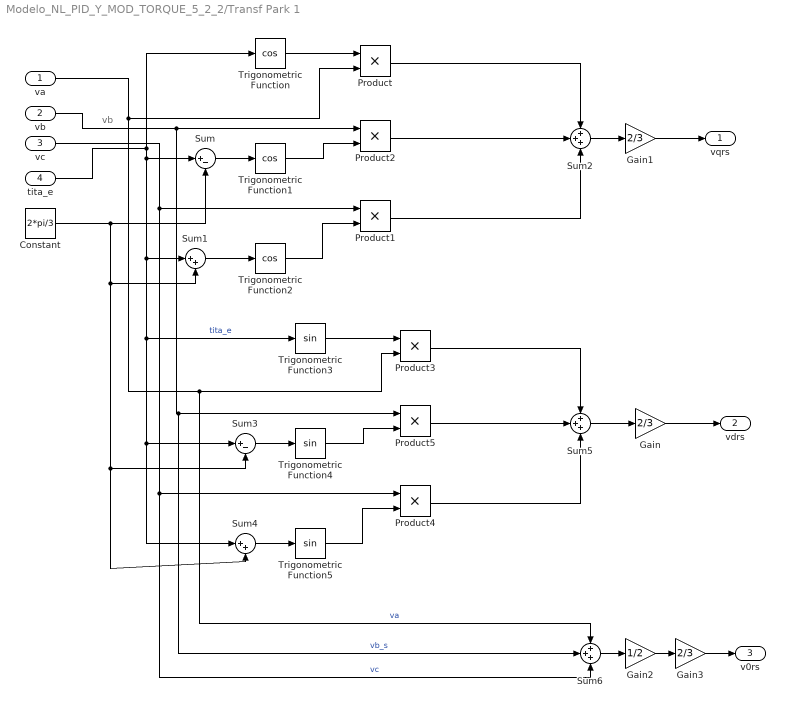
== system Modelo_NL_PID_Y_MOD_TORQUE_5_2_2/Transf Park 1 ==
  note: vb
  "va " : Inport
  vb : Inport  Port=2
  vc : Inport  Port=3
  tita_e : Inport  Port=4
  Constant : Constant  Value=2*pi/3
  Gain : Gain  Gain=2/3
  Gain1 : Gain  Gain=2/3
  Gain2 : Gain  Gain=1/2
  Gain3 : Gain  Gain=2/3
  Product{,1..5} (6 alike) : Product
  Sum : Sum  Inputs=|+-
  Sum1 : Sum  Inputs=|++
  Sum2 : Sum  Inputs=+++
  Sum3 : Sum  Inputs=|+-
  Sum4 : Sum  Inputs=|++
  Sum5 : Sum  Inputs=+++
  Sum6 : Sum  Inputs=+++
  Trigonometric Function : Trigonometry  Operator=cos
  Trigonometric Function1 : Trigonometry  Operator=cos
  Trigonometric Function2 : Trigonometry  Operator=cos
  Trigonometric Function3 : Trigonometry
  Trigonometric Function4 : Trigonometry
  Trigonometric Function5 : Trigonometry
  vqrs : Outport
  "vdrs " : Outport  Port=2
  "v0rs " : Outport  Port=3
  wires:
  tita_e/1 -> Sum1/1, Trigonometric Function3/1, Sum3/1, Sum4/1, Sum/1, Trigonometric Function/1  "tita_e"
  Trigonometric Function/1 -> Product/1
  "va "/1 -> Sum6/1, Product3/2, Product/2  "va"
  Constant/1 -> Sum4/2, Sum3/2, Sum1/2, Sum/2
  Sum/1 -> Trigonometric Function1/1
  Sum1/1 -> Trigonometric Function2/1
  Trigonometric Function1/1 -> Product2/2
  Trigonometric Function2/1 -> Product1/2
  vb/1 -> Sum6/2, Product5/1, Product2/1  "vb_s"
  vc/1 -> Sum6/3, Product4/1, Product1/1  "vc"
  Product/1 -> Sum2/1
  Product2/1 -> Sum2/2
  Sum2/1 -> Gain1/1
  Trigonometric Function5/1 -> Product4/2
  Trigonometric Function3/1 -> Product3/1
  Sum4/1 -> Trigonometric Function5/1
  Sum3/1 -> Trigonometric Function4/1
  Trigonometric Function4/1 -> Product5/2
  Product3/1 -> Sum5/1
  Product5/1 -> Sum5/2
  Product4/1 -> Sum5/3
  Sum5/1 -> Gain/1
  Product1/1 -> Sum2/3
  Gain/1 -> "vdrs "/1
  Gain1/1 -> vqrs/1
  Sum6/1 -> Gain2/1
  Gain3/1 -> "v0rs "/1
  Gain2/1 -> Gain3/1

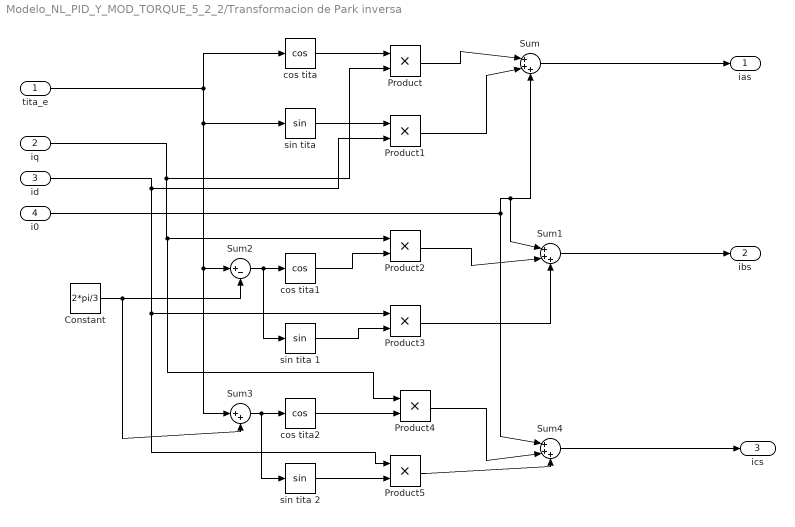
== system Modelo_NL_PID_Y_MOD_TORQUE_5_2_2/Transformacion de Park inversa  ==
  tita_e : Inport
  iq : Inport  Port=2
  id : Inport  Port=3
  i0 : Inport  Port=4
  Constant : Constant  Value=2*pi/3
  Product{,1..5} (6 alike) : Product
  Sum : Sum  Inputs=|+++
  Sum1 : Sum  Inputs=|+++
  Sum2 : Sum  Inputs=|+-
  Sum3 : Sum  Inputs=|++
  Sum4 : Sum  Inputs=|+++
  cos tita : Trigonometry  Operator=cos
  cos tita1 : Trigonometry  Operator=cos
  cos tita2 : Trigonometry  Operator=cos
  "sin tita " : Trigonometry
  sin tita 1 : Trigonometry
  sin tita 2 : Trigonometry
  ias : Outport
  ibs : Outport  Port=2
  "ics " : Outport  Port=3
  wires:
  tita_e/1 -> Sum3/1, Sum2/1, "sin tita "/1, cos tita/1
  iq/1 -> Product4/1, Product2/1, Product/2
  cos tita/1 -> Product/1
  "sin tita "/1 -> Product1/1
  id/1 -> Product5/1, Product3/1, Product1/2
  Product/1 -> Sum/1
  Product1/1 -> Sum/2
  Sum/1 -> ias/1
  i0/1 -> Sum1/1, Sum/3, Sum4/1
  cos tita1/1 -> Product2/2
  sin tita 1/1 -> Product3/2
  Product3/1 -> Sum1/3
  Product2/1 -> Sum1/2
  Sum1/1 -> ibs/1
  Constant/1 -> Sum3/2, Sum2/2
  Sum2/1 -> sin tita 1/1, cos tita1/1
  Sum3/1 -> sin tita 2/1, cos tita2/1
  cos tita2/1 -> Product4/2
  sin tita 2/1 -> Product5/2
  Product5/1 -> Sum4/3
  Product4/1 -> Sum4/2
  Sum4/1 -> "ics "/1

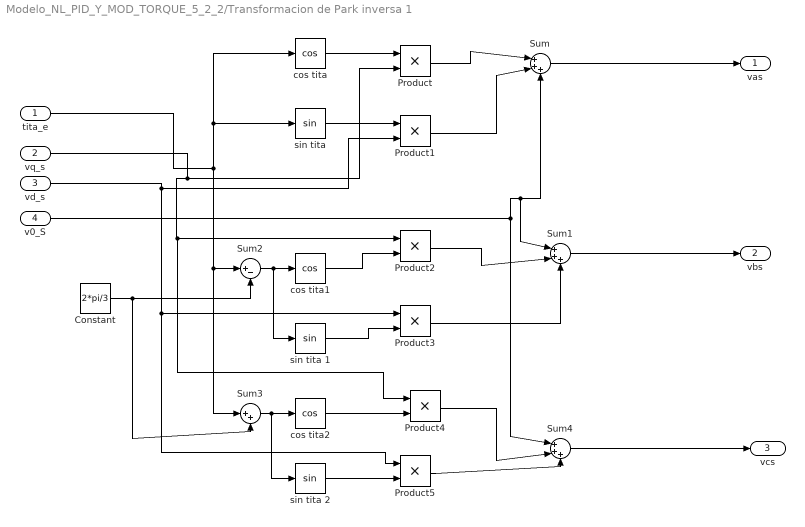
== system Modelo_NL_PID_Y_MOD_TORQUE_5_2_2/Transformacion de Park inversa 1 ==
  tita_e : Inport
  vq_s : Inport  Port=2
  vd_s : Inport  Port=3
  "v0_S " : Inport  Port=4
  Constant : Constant  Value=2*pi/3
  Product{,1..5} (6 alike) : Product
  Sum : Sum  Inputs=|+++
  Sum1 : Sum  Inputs=|+++
  Sum2 : Sum  Inputs=|+-
  Sum3 : Sum  Inputs=|++
  Sum4 : Sum  Inputs=|+++
  cos tita : Trigonometry  Operator=cos
  cos tita1 : Trigonometry  Operator=cos
  cos tita2 : Trigonometry  Operator=cos
  "sin tita " : Trigonometry
  sin tita 1 : Trigonometry
  sin tita 2 : Trigonometry
  vas : Outport
  vbs : Outport  Port=2
  "vcs " : Outport  Port=3
  wires:
  tita_e/1 -> Sum3/1, Sum2/1, cos tita/1, "sin tita "/1
  vq_s/1 -> Product4/1, Product2/1, Product/2
  cos tita/1 -> Product/1
  "sin tita "/1 -> Product1/1
  vd_s/1 -> Product5/1, Product3/1, Product1/2
  Product/1 -> Sum/1
  Product1/1 -> Sum/2
  Sum/1 -> vas/1
  "v0_S "/1 -> Sum1/1, Sum/3, Sum4/1
  cos tita1/1 -> Product2/2
  sin tita 1/1 -> Product3/2
  Product3/1 -> Sum1/3
  Product2/1 -> Sum1/2
  Sum1/1 -> vbs/1
  Constant/1 -> Sum3/2, Sum2/2
  Sum2/1 -> sin tita 1/1, cos tita1/1
  Sum3/1 -> sin tita 2/1, cos tita2/1
  cos tita2/1 -> Product4/2
  sin tita 2/1 -> Product5/2
  Product5/1 -> Sum4/3
  Product4/1 -> Sum4/2
  Sum4/1 -> "vcs "/1

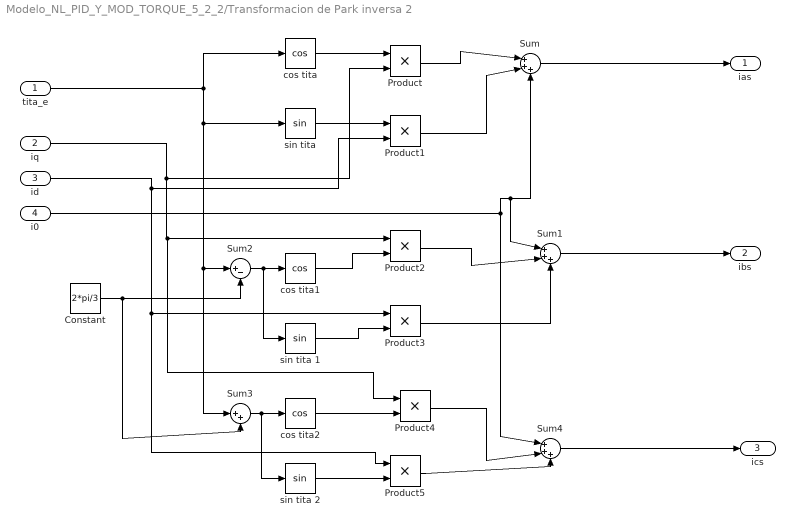
== system Modelo_NL_PID_Y_MOD_TORQUE_5_2_2/Transformacion de Park inversa 2 ==
  tita_e : Inport
  iq : Inport  Port=2
  id : Inport  Port=3
  i0 : Inport  Port=4
  Constant : Constant  Value=2*pi/3
  Product{,1..5} (6 alike) : Product
  Sum : Sum  Inputs=|+++
  Sum1 : Sum  Inputs=|+++
  Sum2 : Sum  Inputs=|+-
  Sum3 : Sum  Inputs=|++
  Sum4 : Sum  Inputs=|+++
  cos tita : Trigonometry  Operator=cos
  cos tita1 : Trigonometry  Operator=cos
  cos tita2 : Trigonometry  Operator=cos
  "sin tita " : Trigonometry
  sin tita 1 : Trigonometry
  sin tita 2 : Trigonometry
  ias : Outport
  ibs : Outport  Port=2
  "ics " : Outport  Port=3
  wires:
  tita_e/1 -> Sum3/1, Sum2/1, "sin tita "/1, cos tita/1
  iq/1 -> Product4/1, Product2/1, Product/2
  cos tita/1 -> Product/1
  "sin tita "/1 -> Product1/1
  id/1 -> Product5/1, Product3/1, Product1/2
  Product/1 -> Sum/1
  Product1/1 -> Sum/2
  Sum/1 -> ias/1
  i0/1 -> Sum1/1, Sum/3, Sum4/1
  cos tita1/1 -> Product2/2
  sin tita 1/1 -> Product3/2
  Product3/1 -> Sum1/3
  Product2/1 -> Sum1/2
  Sum1/1 -> ibs/1
  Constant/1 -> Sum3/2, Sum2/2
  Sum2/1 -> sin tita 1/1, cos tita1/1
  Sum3/1 -> sin tita 2/1, cos tita2/1
  cos tita2/1 -> Product4/2
  sin tita 2/1 -> Product5/2
  Product5/1 -> Sum4/3
  Product4/1 -> Sum4/2
  Sum4/1 -> "ics "/1

== system Modelo_NL_PID_Y_MOD_TORQUE_5_2_2/Transformacion de Park inversa 3 ==
  tita_e : Inport
  vq_s : Inport  Port=2
  vd_s : Inport  Port=3
  "v0_S " : Inport  Port=4
  Constant : Constant  Value=2*pi/3
  Product{,1..5} (6 alike) : Product
  Sum : Sum  Inputs=|+++
  Sum1 : Sum  Inputs=|+++
  Sum2 : Sum  Inputs=|+-
  Sum3 : Sum  Inputs=|++
  Sum4 : Sum  Inputs=|+++
  cos tita : Trigonometry  Operator=cos
  cos tita1 : Trigonometry  Operator=cos
  cos tita2 : Trigonometry  Operator=cos
  "sin tita " : Trigonometry
  sin tita 1 : Trigonometry
  sin tita 2 : Trigonometry
  vas : Outport
  vbs : Outport  Port=2
  "vcs " : Outport  Port=3
  wires:
  tita_e/1 -> Sum3/1, Sum2/1, cos tita/1, "sin tita "/1
  vq_s/1 -> Product4/1, Product2/1, Product/2
  cos tita/1 -> Product/1
  "sin tita "/1 -> Product1/1
  vd_s/1 -> Product5/1, Product3/1, Product1/2
  Product/1 -> Sum/1
  Product1/1 -> Sum/2
  Sum/1 -> vas/1
  "v0_S "/1 -> Sum1/1, Sum/3, Sum4/1
  cos tita1/1 -> Product2/2
  sin tita 1/1 -> Product3/2
  Product3/1 -> Sum1/3
  Product2/1 -> Sum1/2
  Sum1/1 -> vbs/1
  Constant/1 -> Sum3/2, Sum2/2
  Sum2/1 -> sin tita 1/1, cos tita1/1
  Sum3/1 -> sin tita 2/1, cos tita2/1
  cos tita2/1 -> Product4/2
  sin tita 2/1 -> Product5/2
  Product5/1 -> Sum4/3
  Product4/1 -> Sum4/2
  Sum4/1 -> "vcs "/1

== system Modelo_NL_PID_Y_MOD_TORQUE_5_2_2/Velocidad trapezoidal ==
  Bus Creator : BusCreator  Tag=Bus Creator  Inputs=1
  FromWs : FromWorkspace  Tag=STV FromWs  VariableName=tuvar  SampleTime=0
      SigBuilderData=|
      | common.afterFinalStr = 'Extrapolate'
      | common.sampleTime = 0
      | dataSet.timeRange = [0 25]
      | dataSet.name = 'Group 1'
      | sbobj.Groups.Name = 'Group 1'
      | sbobj.Groups.Signals.Name = 'Signal 1'
      | sbobj.Groups.Signals.XData = [0 5 5.497 9.502 10 15 15.49 19.497 20 25]
      | sbobj.Groups.Signals.YData = [0 0 380 380 0 0 -380 -380 0 0]
      | sbobj.Groups.TimeRange = [0 25]
  Subsystem : Subsystem
  Bus : Outport
  wires:
  FromWs/1 -> Subsystem/1(In1)
  Bus Creator/1 -> Bus/1
  Subsystem/1(Signal 1) -> Bus Creator/1  "Signal 1"

== system Modelo_NL_PID_Y_MOD_TORQUE_5_2_2/Velocidad trapezoidal1 ==
  Bus Creator : BusCreator  Tag=Bus Creator  Inputs=1
  FromWs : FromWorkspace  Tag=STV FromWs  VariableName=tuvar  SampleTime=0
      SigBuilderData=|
      | common.afterFinalStr = 'Extrapolate'
      | common.sampleTime = 0
      | dataSet.timeRange = [0 25]
      | dataSet.name = 'Group 1'
      | sbobj.Groups.Name = 'Group 1'
      | sbobj.Groups.Signals.Name = 'Signal 1'
      | sbobj.Groups.Signals.XData = [0 5 5.497 9.502 10 15 15.49 19.497 20 25]
      | sbobj.Groups.Signals.YData = [0 0 380 380 0 0 -380 -380 0 0]
      | sbobj.Groups.TimeRange = [0 25]
  Subsystem : Subsystem
  Bus : Outport
  wires:
  FromWs/1 -> Subsystem/1(In1)
  Bus Creator/1 -> Bus/1
  Subsystem/1(Signal 1) -> Bus Creator/1  "Signal 1"

== system Modelo_NL_PID_Y_MOD_TORQUE_5_2_2/Modelo físico (subsistema electromagnético + mecanico)/Eq 1 ==
  vqrs : Inport
  "Producto 1 " : Inport  Port=2
  Rs : Inport  Port=3
  Gain : Gain  Gain=1/Lq
  Integrator : Integrator
  Product : Product
  Sum : Sum  Inputs=+--
  "iqrs " : Outport
  wires:
  Gain/1 -> Integrator/1
  Sum/1 -> Gain/1
  vqrs/1 -> Sum/1
  Product/1 -> Sum/2
  "Producto 1 "/1 -> Sum/3
  Integrator/1 -> Product/1, "iqrs "/1  "i_qs"
  Rs/1 -> Product/2

== system Modelo_NL_PID_Y_MOD_TORQUE_5_2_2/Modelo físico (subsistema electromagnético + mecanico)/Eq 2  ==
  "vdrs " : Inport
  "Producto 2 " : Inport  Port=2
  Rs 1 : Inport  Port=3
  Gain2 : Gain  Gain=1/Ld
  Integrator1 : Integrator
  Product : Product
  Sum1 : Sum  Inputs=|+-+
  "idrs " : Outport
  wires:
  "Producto 2 "/1 -> Sum1/3
  Gain2/1 -> Integrator1/1
  Product/1 -> Sum1/2
  Sum1/1 -> Gain2/1
  Integrator1/1 -> Product/1, "idrs "/1  "i_ds"
  "vdrs "/1 -> Sum1/1
  Rs 1/1 -> Product/2

== system Modelo_NL_PID_Y_MOD_TORQUE_5_2_2/Modelo físico (subsistema electromagnético + mecanico)/Eq 3 ==
  "v0rs " : Inport
  Rs 1 : Inport  Port=2
  Gain12 : Gain
  Integrator5 : Integrator
  Producto 1 : Product
  Sum4 : Sum  Inputs=|++
  "i0rs " : Outport
  wires:
  Gain12/1 -> Integrator5/1
  Sum4/1 -> Gain12/1
  Producto 1/1 -> Sum4/2
  "v0rs "/1 -> Sum4/1
  Integrator5/1 -> Producto 1/1, "i0rs "/1  "i_0s"

== system Modelo_NL_PID_Y_MOD_TORQUE_5_2_2/Modelo físico (subsistema electromagnético + mecanico)/Signal Builder ==
  Demux : Demux  Tag=STV Demux  Outputs=1
  FromWs : FromWorkspace  Tag=STV FromWs  VariableName=tuvar  SampleTime=0
      SigBuilderData=|
      | common.afterFinalStr = 'Extrapolate'
      | common.sampleTime = 0
      | dataSet.timeRange = [0 2]
      | dataSet.name = 'Group 1'
      | sbobj.Groups.Name = 'Group 1'
      | sbobj.Groups.Signals.Name = 'Signal 2'
      | sbobj.Groups.Signals.XData = [0 0.3 0.3 0.5 0.5 0.9 0.9 2]
      | sbobj.Groups.Signals.YData = [0 0 0.02 0.02 -0.02 -0.02 0 0]
      | sbobj.Groups.TimeRange = [0 2]
  Signal 2 : Outport  Tag=STV Outport
  wires:
  FromWs/1 -> Demux/1
  Demux/1 -> Signal 2/1

== system Modelo_NL_PID_Y_MOD_TORQUE_5_2_2/Modelo físico (subsistema electromagnético + mecanico)/Subsistema mecánico ==
  "Tleq " : Inport
  "Tmotor " : Inport  Port=2
  Gain6 : Gain  Gain=1/Jeq
  Gain8 : Gain  Gain=beq
  Integrator3 : Integrator
  Integrator4 : Integrator
  Sum3 : Sum  Inputs=-+-
  "tita_m " : Outport
  "wm " : Outport  Port=2
  Tm : Outport  Port=3
  wires:
  Integrator3/1 -> "tita_m "/1
  Integrator4/1 -> Gain8/1, "wm "/1, Integrator3/1
  Sum3/1 -> Tm/1, Gain6/1
  Gain6/1 -> Integrator4/1
  Gain8/1 -> Sum3/3
  "Tleq "/1 -> Sum3/1
  "Tmotor "/1 -> Sum3/2

== system Modelo_NL_PID_Y_MOD_TORQUE_5_2_2/Modelo físico (subsistema electromagnético + mecanico)1/Eq 1 ==
  vqrs : Inport
  "Producto 1 " : Inport  Port=2
  Rs : Inport  Port=3
  Gain : Gain  Gain=1/Lq
  Integrator : Integrator
  Product : Product
  Sum : Sum  Inputs=+--
  "iqrs " : Outport
  wires:
  Gain/1 -> Integrator/1
  Sum/1 -> Gain/1
  vqrs/1 -> Sum/1
  Product/1 -> Sum/2
  "Producto 1 "/1 -> Sum/3
  Integrator/1 -> Product/1, "iqrs "/1  "i_qs"
  Rs/1 -> Product/2

== system Modelo_NL_PID_Y_MOD_TORQUE_5_2_2/Modelo físico (subsistema electromagnético + mecanico)1/Eq 2  ==
  "vdrs " : Inport
  "Producto 2 " : Inport  Port=2
  Rs 1 : Inport  Port=3
  Gain2 : Gain  Gain=1/Ld
  Integrator1 : Integrator
  Product : Product
  Sum1 : Sum  Inputs=|+-+
  "idrs " : Outport
  wires:
  "Producto 2 "/1 -> Sum1/3
  Gain2/1 -> Integrator1/1
  Product/1 -> Sum1/2
  Sum1/1 -> Gain2/1
  Integrator1/1 -> Product/1, "idrs "/1  "i_ds"
  "vdrs "/1 -> Sum1/1
  Rs 1/1 -> Product/2

== system Modelo_NL_PID_Y_MOD_TORQUE_5_2_2/Modelo físico (subsistema electromagnético + mecanico)1/Eq 3 ==
  "v0rs " : Inport
  Rs 1 : Inport  Port=2
  Gain12 : Gain
  Integrator5 : Integrator
  Producto 1 : Product
  Sum4 : Sum  Inputs=|++
  "i0rs " : Outport
  wires:
  Gain12/1 -> Integrator5/1
  Sum4/1 -> Gain12/1
  Producto 1/1 -> Sum4/2
  "v0rs "/1 -> Sum4/1
  Integrator5/1 -> Producto 1/1, "i0rs "/1  "i_0s"

== system Modelo_NL_PID_Y_MOD_TORQUE_5_2_2/Modelo físico (subsistema electromagnético + mecanico)1/Signal Builder ==
  Demux : Demux  Tag=STV Demux  Outputs=1
  FromWs : FromWorkspace  Tag=STV FromWs  VariableName=tuvar  SampleTime=0
      SigBuilderData=|
      | common.afterFinalStr = 'Extrapolate'
      | common.sampleTime = 0
      | dataSet.timeRange = [0 2]
      | dataSet.name = 'Group 1'
      | sbobj.Groups.Name = 'Group 1'
      | sbobj.Groups.Signals.Name = 'Signal 2'
      | sbobj.Groups.Signals.XData = [0 0.3 0.3 0.5 0.5 0.9 0.9 2]
      | sbobj.Groups.Signals.YData = [0 0 0.02 0.02 -0.02 -0.02 0 0]
      | sbobj.Groups.TimeRange = [0 2]
  Signal 2 : Outport  Tag=STV Outport
  wires:
  FromWs/1 -> Demux/1
  Demux/1 -> Signal 2/1

== system Modelo_NL_PID_Y_MOD_TORQUE_5_2_2/Modelo físico (subsistema electromagnético + mecanico)1/Subsistema mecánico ==
  "Tleq " : Inport
  "Tmotor " : Inport  Port=2
  Gain6 : Gain  Gain=1/Jeq
  Gain8 : Gain  Gain=beq
  Integrator3 : Integrator
  Integrator4 : Integrator
  Sum3 : Sum  Inputs=-+-
  "tita_m " : Outport
  "wm " : Outport  Port=2
  Tm : Outport  Port=3
  wires:
  Integrator3/1 -> "tita_m "/1
  Integrator4/1 -> Gain8/1, "wm "/1, Integrator3/1
  Sum3/1 -> Tm/1, Gain6/1
  Gain6/1 -> Integrator4/1
  Gain8/1 -> Sum3/3
  "Tleq "/1 -> Sum3/1
  "Tmotor "/1 -> Sum3/2

== system Modelo_NL_PID_Y_MOD_TORQUE_5_2_2/Posicion trapezoidal/Subsystem ==
  In1 : Inport
  Demux : Demux  Tag=STV Demux  Outputs=1
  Signal 2 : Outport  Tag=STV Outport
  wires:
  In1/1 -> Demux/1
  Demux/1 -> Signal 2/1

== system Modelo_NL_PID_Y_MOD_TORQUE_5_2_2/Posicion trapezoidal1/Subsystem ==
  In1 : Inport
  Demux : Demux  Tag=STV Demux  Outputs=1
  Signal 2 : Outport  Tag=STV Outport
  wires:
  In1/1 -> Demux/1
  Demux/1 -> Signal 2/1

== system Modelo_NL_PID_Y_MOD_TORQUE_5_2_2/Velocidad trapezoidal/Subsystem ==
  In1 : Inport
  Demux : Demux  Tag=STV Demux  Outputs=1
  Signal 1 : Outport  Tag=STV Outport
  wires:
  In1/1 -> Demux/1
  Demux/1 -> Signal 1/1

== system Modelo_NL_PID_Y_MOD_TORQUE_5_2_2/Velocidad trapezoidal1/Subsystem ==
  In1 : Inport
  Demux : Demux  Tag=STV Demux  Outputs=1
  Signal 1 : Outport  Tag=STV Outport
  wires:
  In1/1 -> Demux/1
  Demux/1 -> Signal 1/1
